simulink subsystem "FCS_In"  (R2025a)
settings: Solver=VariableStepAuto  StartTime=0.0  StopTime=10.0  RelTol=1e-3
settings Model: Creator=gurt1  LastModifiedBy=17036

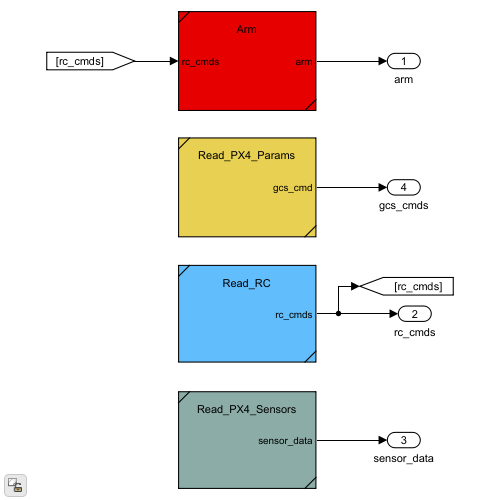
[thumbnail: Simulink's stored preview of the top-level diagram]
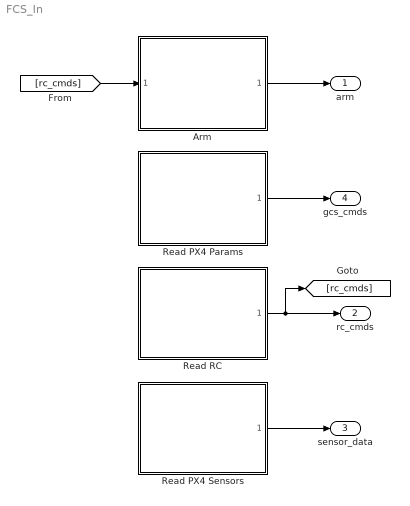
== system FCS_In ==
  Arm : Subsystem  ReferencedSubsystem=Arm
  Read PX4 Params : Subsystem  ReferencedSubsystem=Read_PX4_Params
  Read PX4 Sensors : Subsystem  ReferencedSubsystem=Read_PX4_Sensors
  Read RC : Subsystem  ReferencedSubsystem=Read_RC
  arm : Outport
  rc_cmds : Outport  Port=2
  sensor_data : Outport  Port=3
  gcs_cmds : Outport  Port=4
  wires:
  Read RC/1 -> rc_cmds/1, [rc_cmds]
  Read PX4 Params/1 -> gcs_cmds/1
  Read PX4 Sensors/1 -> sensor_data/1
  Arm/1 -> arm/1
  [rc_cmds] -> Arm/1
